simulink library "SignalGeneratorLib"  (R2022b)
settings: Solver=VariableStepAuto  StartTime=0.0  StopTime=10.0  RelTol=1e-3
values from neighbouring files (symbols this model uses):
  cycles_per_step = 10    [chimes_init.m]
  default_time = 1    [chimes_init.m]
  end_freq_Hz = 1000    [chimes_init.m]
  log_sweep_ON = 1    [chimes_init.m]
  multitone_channel_map = 3    [chimes_init.m]
  multitone_ON = 6    [chimes_init.m]
  Nch = 4    [ChimeControlConfig.m]    (also in chimes_init.m = 1)
  nch = Nch    (= 1)    [chimes_init.m]
  Num_Multitone_channels = 1    [chimes_init.m]
  NumTones = 3    [SignalGeneratorConfig.m]    (also in chimes_init.m)
  old_sweep_ON = 3    [chimes_init.m]
  random_noise = 0.5    [chimes_init.m]
  random_noise_ON = 4    [chimes_init.m]
  sawtooth_mode_ON = 5    [chimes_init.m]
  sineTable = 0.99 * sin( 2 * pi * time_values )    [chimes_init.m]
  start_freq_Hz = 50    [chimes_init.m]
  start_frequencies = 240    [chimes_init.m]
  start_phase = 0    [chimes_init.m]
  start_phase_rad = [0 pi/2 pi]    [chimes_init.m]
  steps = 5    [chimes_init.m]
  sweep_time_sec = 0.25    [chimes_init.m]
  Tone_freq_Hz = [440 550 750]    [chimes_init.m]
  ToneGains = [1 1 1]    [chimes_init.m]
  tuneTop_time = 0    [chimes_init.m]
undefined symbols (not defined in the file or in its folder): end_freq_Hz_phaseDetector, linear_sweep_ON_phaseDetector, Numch, start_freq_Hz_phaseDetector, start_phase_rad_LinearSweep_phaseDetector, sweep_time_sec_phaseDetector, sys_defs
libraries: SignalGeneratorLibBtc x6
settings Model: Creator=sc48041  LastModifiedBy=kl13806
settings SolverCC: AlgebraicLoopSolver=TrustRegion
settings DebuggingCC: UnconnectedInputMsg=warning  UnconnectedOutputMsg=warning  UnconnectedLineMsg=warning  SFMachineParentedDataDiag=warning
settings ModelReferenceCC: EnableRefExpFcnMdlSchedulingChecks=on
settings RTWCC: DLArmComputeVersion=19.05

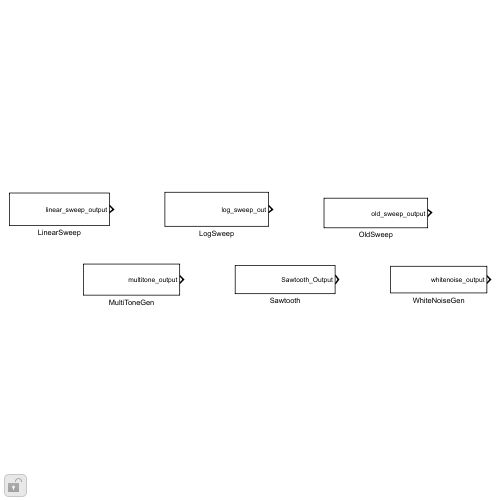
[thumbnail: Simulink's stored preview of the top-level diagram]
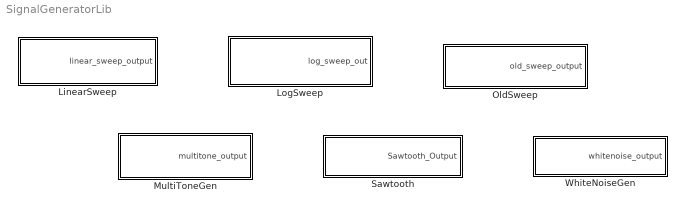
== system SignalGeneratorLib ==
  LinearSweep : Subsystem  mask{Fs_Hz=sys_defs.Fs_Hz, frameSize_samples=sys_defs.frameSize_samples, sineTableLength=sys_defs.sineTableLength, sineTable=sys_defs.sineTable, Nch=Numch, linear_sweep_ON=linear_sweep_ON_phaseDetector, start_freq_Hz=start_freq_Hz_phaseDetector, end_freq_Hz=end_freq_Hz_phaseDetector, sweep_time_sec=sweep_time_sec_phaseDetector, start_phase_rad=start_phase_rad_LinearSweep_phaseDetector}
      mask init:
      | blkh = gcbh;
      | % Copy discrete mask parameters into a classdef object
      | InnerLinkConfig = LinearSweepConfig;
      | InnerLinkConfig.FsHz = Fs_Hz;
      | InnerLinkConfig.FrameSizeSamples = frameSize_samples;
      | InnerLinkConfig.SineTableLength = sineTableLength;
      | InnerLinkConfig.SineTable = sineTable;
      | InnerLinkConfig.NumChannel = Nch;
      | InnerLinkConfig.LinearSweepOn = linear_sweep_ON;
      | InnerLinkConfig.StartFreqHz = start_freq_Hz;
      | InnerLinkConfig.EndFreqHz = end_freq_Hz;
      | InnerLinkConfig.SweepTimeSec = sweep_time_sec;
      | InnerLinkConfig.StartPhaseRad = start_phase_rad;
  LogSweep : Subsystem  mask{Fs_Hz=sys_defs.Fs_Hz, frameSize_samples=sys_defs.frameSize_samples, sineTableLength=sys_defs.sineTableLength, sineTable=sys_defs.sineTable, Nch=Nch, log_sweep_ON=log_sweep_ON, start_freq_Hz=start_freq_Hz, end_freq_Hz=end_freq_Hz, sweep_time_sec=sweep_time_sec, start_phase_rad=start_phase_rad}
      mask init:
      | blkh = gcbh;
      | % Copy discrete mask parameters into a classdef object
      | InnerLinkConfig = LogSweepConfig;
      | InnerLinkConfig.FsHz = Fs_Hz;
      | InnerLinkConfig.FrameSizeSamples = frameSize_samples;
      | InnerLinkConfig.SineTableLength = sineTableLength;
      | InnerLinkConfig.SineTable = sineTable;
      | InnerLinkConfig.NumChannel = Nch;
      | InnerLinkConfig.LogSweepOn = log_sweep_ON;
      | InnerLinkConfig.StartFreqHz = start_freq_Hz;
      | InnerLinkConfig.EndFreqHz = end_freq_Hz;
      | InnerLinkConfig.SweepTimeSec = sweep_time_sec;
      | InnerLinkConfig.StartPhaseRad = start_phase_rad;
  MultiToneGen : Subsystem  mask(Bose Multi tone){Fs_Hz=sys_defs.Fs_Hz, frameSize_samples=sys_defs.frameSize_samples, sineTableLength=sys_defs.sineTableLength, sineTable=sineTable, multitone_ON=multitone_ON, multitone_channel_map=multitone_channel_map, Num_Multitone_channels=Num_Multitone_channels, NumTones=NumTones, Tone_freq_Hz=Tone_freq_Hz, start_phase_rad=start_phase_rad, ToneGains=ToneGains}
      mask help:
      | This block is used for generating a multi channel multi tone signal by using a sinusoid generator that supports arbirtrary frequencies by interpolating from a sine table.
      |
      | multitone_ON   :
      | Mode selection for enable/disable of multitone signal
      | 0 = Off
      | 6 = Multitone Signal
      | Example : multitone_ON =6 enables multi tone signal, multitone_ON=0 disables the multi tone signal
      |
      | multitone_channel_map   :
      | Number of tones in each channel
      | Example : multitone_channel_map = [2 3] , Indicates that there are 5 tones which needs to be mapped to 2 output channels.
      | 1st output channel has 2 tones summed up and 2nd output channel has 3 tones summed up.
      |
      | Num_Multitone_channels :
      | Indicates that there are multiple output channels ,each channel has multitone signal.
      | Example : Num_Multitone_channels=1 and multitone_channel_map =[4] means there is 1 output channel having 4 tones summed up.
      |
      | NumTones :
      | Total Number of tones
      | Example : NumTones=4 and multitone_channel_map =[4] indicates there is 1 output channel having  4 tones summed up.
      |
      | Tone_freq_Hz :
      | Vector of Frequency values in Hz for each Tone
      | Example : Tone_freq_Hz=[100 200 300]  means there are 3 tones of 100 ,200 and 300 Hz which may be assigned to 1 output channel or multiple channels
      | based on multitone_channel_map.
      | If multitone_channel_map=[1 2],this means 1st output channel will have only 100 Hz output i.e single tone signal.
      | and 2nd output channel will have 200 Hz and 300 Hz tones summed up.
      |
      | start_phase_rad :
      | Vector of Starting phase values in radians for each tone
      | Example : start_phase_rad=[0 pi/2 pi]
      |
      | ToneGains :
      | Vector of Gain values for each tone
      | Example : start_phase_rad=[0 0.25 0.5], multitone_channel_map=[3] means there is 1 output channel with 3 tones summed up and total gain observed
      | at output channel will be a sum close to 0.75
      mask init:
      | blkh = gcbh;
      | % Copy discrete mask parameters into a classdef object
      | InnerLinkConfig = MultiToneGenConfig;
      | InnerLinkConfig.FsHz = Fs_Hz;
      | InnerLinkConfig.FrameSizeSamples = frameSize_samples;
      | InnerLinkConfig.SineTableLength = sineTableLength;
      | InnerLinkConfig.SineTable = sineTable;
      | InnerLinkConfig.MultitoneOn = multitone_ON;
      | InnerLinkConfig.MultitoneChannelMap = multitone_channel_map;
      | InnerLinkConfig.NumMultitoneChannels = Num_Multitone_channels;
      | InnerLinkConfig.NumTones = NumTones;
      | InnerLinkConfig.ToneFreqHz = Tone_freq_Hz;
      | InnerLinkConfig.StartPhaseRad = start_phase_rad;
      | InnerLinkConfig.ToneGains = ToneGains;
      mask Help:
      | Configuration Parameters:
      | 
      |   multitone_ON
      |                         : mode: Vector of modes for each channel's operation
      | 						  0 = Off
      | 						  1 = Logarithmic sine sweep
      | 						  2 = Linear sine sweep
      | 						  3 = Old style sine sweep
      | 						  4 = Random noise
      | 						  5 = Sawtooth wave (Does not support sweep)
      | 						  6 = Multitone Signal
      | 						 Example : multitone_ON =6
      | 
      |   multitone_channel_map
      |                         : Number of tones in each channel
      | 						Example : multitone_channel_map = [2 3] , Indicates that there are 5 tones which needs to be mapped to 2 output channels.
      | 						1st output channel has 2 tones summed up and 2nd output channel has 3 tones summed up.
      |   Num_Multitone_channels
      |                         : Indicates that there are multiple output channels ,each channel has multitone signal.
      | 						Example : Num_Multitone_channels=1 and multitone_channel_map =[4] means there is 1 output channel having 4 tones summed up.
      |   NumTones
      |                         : Total Number of tones
      | 						Example : NumTones=4 and multitone_channel_map =[4] indicates there is 1 output channel having  4 tones summed up.
      |   Tone_freq_Hz
      |                         : Vector of Frequency values in Hz for each Tone
      | 						Example : Tone_freq_Hz=[100 200 300]  means there are 3 tones of 100 ,200 and 300 Hz which may be assigned to 1 output channel or multiple channels
      | 						based on multitone_channel_map.
      | 						If multitone_channel_map=[1 2],
      | 						this means 1st output channel will have only 100 Hz output i.e single tone signal.
      | 						and 2nd output channel will have 200 Hz and 300 Hz tones summed up.
      |   start_phase_rad
      |                         : Vector of Starting phase values in radians for each tone
      | 						Example : start_phase_rad=[0 pi/2 pi]
      |   ToneGains
      |                         : Vector of Gain values for each tone
      | 						Example : start_phase_rad=[0 0.25 0.5], multitone_channel_map=[3] means there is 1 output channel with 3 tones summed up and total gain observed
      | 						at output channel will be a sum close to 0.75
  OldSweep : Subsystem  mask{Fs_Hz=sys_defs.Fs_Hz, frameSize_samples=sys_defs.frameSize_samples, sineTableLength=sys_defs.sineTableLength, sineTable=sys_defs.sineTable, Nch=Nch, old_sweep_ON=old_sweep_ON, start_freq_Hz=start_freq_Hz, end_freq_Hz=end_freq_Hz, steps=steps, start_phase_rad=start_phase_rad, cycles_per_stepc=cycles_per_step}
      mask prompts: cycles_per_stepc "cycles_per_step"
      mask init:
      | blkh = gcbh;
      | % Copy discrete mask parameters into a classdef object
      | InnerLinkConfig = OldSweepConfig;
      | InnerLinkConfig.FsHz = Fs_Hz;
      | InnerLinkConfig.FrameSizeSamples = frameSize_samples;
      | InnerLinkConfig.SineTableLength = sineTableLength;
      | InnerLinkConfig.SineTable = sineTable;
      | InnerLinkConfig.NumChannel = Nch;
      | InnerLinkConfig.OldSweepOn = old_sweep_ON;
      | InnerLinkConfig.StartFreqHz = start_freq_Hz;
      | InnerLinkConfig.EndFreqHz = end_freq_Hz;
      | InnerLinkConfig.Steps = steps;
      | InnerLinkConfig.StartPhaseRad = start_phase_rad;
      | InnerLinkConfig.CyclesPerStepc = cycles_per_stepc;
  Sawtooth : Subsystem  mask{Fs_Hz=sys_defs.Fs_Hz, frameSize_samples=sys_defs.frameSize_samples, Nch=nch, sawtooth_mode_ON=sawtooth_mode_ON, start_frequencies=start_frequencies, start_phase=start_phase, tuneTop_time=tuneTop_time, default_time=default_time}
      mask init:
      | blkh = gcbh;
      | % Copy discrete mask parameters into a classdef object
      | InnerLinkConfig = SawtoothConfig;
      | InnerLinkConfig.FsHz = Fs_Hz;
      | InnerLinkConfig.FrameSizeSamples = frameSize_samples;
      | InnerLinkConfig.NumChannel = Nch;
      | InnerLinkConfig.SawtoothModeOn = sawtooth_mode_ON;
      | InnerLinkConfig.StartFreqHz = start_frequencies;
      | InnerLinkConfig.StartPhaseRad = start_phase;
      | InnerLinkConfig.DefaultTuneTopTime = tuneTop_time;
      | InnerLinkConfig.DefaultTime = default_time;
  WhiteNoiseGen : Subsystem  mask{Fs_Hz=sys_defs.Fs_Hz, frameSize_samples=sys_defs.frameSize_samples, Nch=nch, random_noise_ON=random_noise_ON, random_noise=random_noise}
      mask init:
      | blkh = gcbh;
      | % Copy discrete mask parameters into a classdef object
      | InnerLinkConfig = WhiteNoiseGenConfig;
      | InnerLinkConfig.FsHz = Fs_Hz;
      | InnerLinkConfig.FrameSizeSamples = frameSize_samples;
      | InnerLinkConfig.NumChannel = Nch;
      | InnerLinkConfig.RandomNoiseOn = random_noise_ON;
      | InnerLinkConfig.RandomNoise = random_noise;

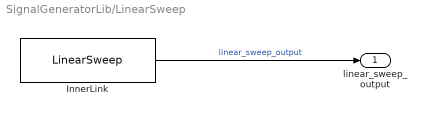
== system SignalGeneratorLib/LinearSweep ==
  InnerLink : SignalGeneratorLibBtc/LinearSweep  Config=InnerLinkConfig  FeatureName=SignalGeneratorLinearSweep
      settings: SourceProductName=Bose Blocklib
  linear_sweep_output : Outport
  wires:
  InnerLink/1 -> linear_sweep_output/1  "linear_sweep_output"

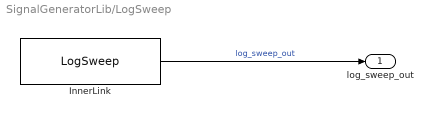
== system SignalGeneratorLib/LogSweep ==
  InnerLink : SignalGeneratorLibBtc/LogSweep  Config=InnerLinkConfig  FeatureName=SignalGeneratorLogSweep
      settings: SourceProductName=Bose Blocklib
  log_sweep_out : Outport
  wires:
  InnerLink/1 -> log_sweep_out/1  "log_sweep_out"

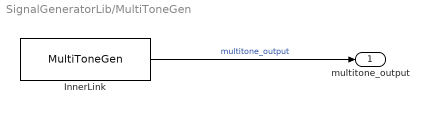
== system SignalGeneratorLib/MultiToneGen ==
  InnerLink : SignalGeneratorLibBtc/MultiToneGen  Config=InnerLinkConfig  FeatureName=SignalGeneratorMultitone
      settings: SourceProductName=Bose Blocklib
  multitone_output : Outport
  wires:
  InnerLink/1 -> multitone_output/1  "multitone_output"

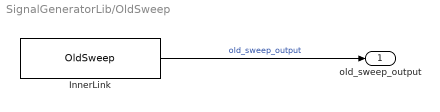
== system SignalGeneratorLib/OldSweep ==
  InnerLink : SignalGeneratorLibBtc/OldSweep  Config=InnerLinkConfig  FeatureName=SignalGeneratorOldSweep
      settings: SourceProductName=Bose Blocklib
  old_sweep_output : Outport
  wires:
  InnerLink/1 -> old_sweep_output/1  "old_sweep_output"

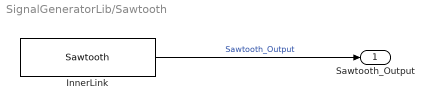
== system SignalGeneratorLib/Sawtooth ==
  InnerLink : SignalGeneratorLibBtc/Sawtooth  Config=InnerLinkConfig  FeatureName=SignalGeneratorSawtooth
      settings: SourceProductName=Bose Blocklib
  Sawtooth_Output : Outport
  wires:
  InnerLink/1 -> Sawtooth_Output/1  "Sawtooth_Output"

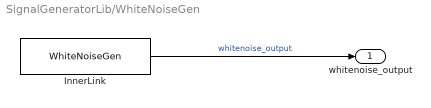
== system SignalGeneratorLib/WhiteNoiseGen ==
  InnerLink : SignalGeneratorLibBtc/WhiteNoiseGen  Config=InnerLinkConfig  FeatureName=SignalGeneratorRandomNoise
      settings: SourceProductName=Bose Blocklib
  whitenoise_output : Outport
  wires:
  InnerLink/1 -> whitenoise_output/1  "whitenoise_output"
